simulink model "gm_inc_enc_v25"  (R2022a)
settings: Solver=FixedStepDiscrete  StartTime=0.0  StopTime=SimulationsDauer  RelTol=1e-3
undefined symbols (not defined in the file or in its folder): DiscIntNeverNeededParam, f_ISR, IncPerTurn, inital_zero_speed_timeout, n_max, OmegaPerOverSampl, Periode, Phase_Delay_A, Phase_Delay_B, PolePair, QuadratureFactor, reciprocal_iterations, T_fpga, T_mech
libraries: hdlsllib x7, hdlmdlgenlib x4, dspsrcs4 x3, dspswit3 x2, spsEdgeDetectorLib x2, simulink_extras x1
(part 2 of 2)

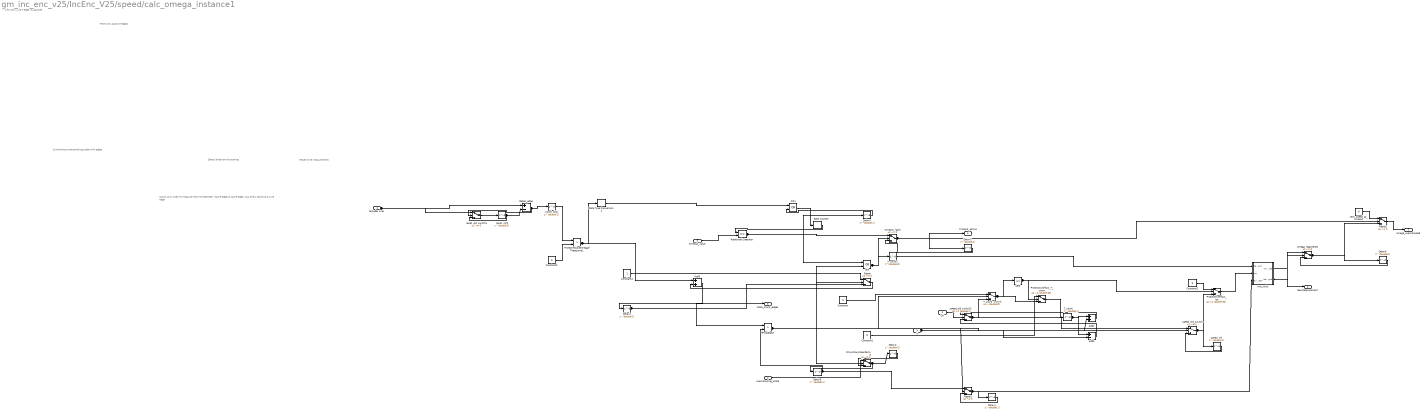
== system gm_inc_enc_v25/IncEnc_V25/speed/calc_omega_instance1 ==
  note: Count up in order to measure the time between "same edge to same edge", e.g. every positive A-Line edge
  note: Reset time measurement
  note: 1 for one cycle if edge recognized
  note: Select direction of counting
  note: Filter only positive edges
  note: Synchronize oversampling state with edges
  Encoder Line : Inport  OutDataTypeStr=boolean  PortDimensions=1  SampleTime=1e-08
  Dir : Inport  Port=2  OutDataTypeStr=fixdt(1, 4, 0)  PortDimensions=1  SampleTime=1e-08
  T : Inport  Port=3  OutDataTypeStr=fixdt(1, 38, 32)  PortDimensions=1  SampleTime=1e-08
  oversampling_state : Inport  Port=4  OutDataTypeStr=uint16  PortDimensions=1  SampleTime=1e-08
  timeout_value : Inport  Port=5  OutDataTypeStr=uint32  PortDimensions=1  SampleTime=1e-08
  32bit counter : hdlsllib/Sources/HDL Counter  CountType=Free running  CountInit=0  CountStep=1  CountMax=inital_zero_speed_timeout  CountFromType=Initial value  CountFrom=0  CountResetPort=on  CountLoadPort=off  CountEnbPort=off  CountDirPort=off  CountHitOutputPort=off  CountDataType=Unsigned  CountWordLen=32  CountFracLen=0  CountSampTime=1
  ABS : Abs  SampleTime=1e-08  OutDataTypeStr=fixdt(1, 38, 32)  SaturateOnIntegerOverflow=off
  Add1 : Sum  AccumDataTypeStr=fixdt(1, 38, 32)  OutDataTypeStr=fixdt(1, 38, 32)  SampleTime=1e-08
  Add2 : Sum  Inputs=+-  AccumDataTypeStr=fixdt(1, 38, 32)  OutDataTypeStr=fixdt(1, 38, 32)  SampleTime=1e-08
  Add3 : Sum  AccumDataTypeStr=int16  OutDataTypeStr=int16  SampleTime=1e-08
  Constant : Constant  Value=0  OutDataTypeStr=fixdt(1, 38, 32)  SampleTime=1e-08
  Constant1 : Constant  Value=0  OutDataTypeStr=fixdt(1, 38, 32)  SampleTime=1e-08
  Constant2 : Constant  Value=0  OutDataTypeStr=fixdt(1, 38, 32)  SampleTime=1e-08
  Constant3 : Constant  Value=0  OutDataTypeStr=int8  SampleTime=1e-08
  Constant4 : Constant  OutDataTypeStr=int8  SampleTime=1e-08
  Data Type Conversion1 : DataTypeConversion  OutDataTypeStr=boolean  SampleTime=1e-08  SaturateOnIntegerOverflow=off  RndMeth=Floor
  Delay{1..6,8} (7 alike) : Delay  DelayLength=double(1)  InitialCondition=0  SampleTime=1e-08
  Detec_edge : Sum  Inputs=+-  AccumDataTypeStr=int8  OutDataTypeStr=int8  SampleTime=1e-08
  IfFinalState : RelationalOperator  Operator=>  OutDataTypeStr=boolean  SampleTime=1e-08  InputSameDT=off
  OR : Logic  Operator=OR  AllPortsSameDT=off  OutDataTypeStr=boolean  SampleTime=1e-08
  OR1 : Logic  Operator=OR  AllPortsSameDT=off  OutDataTypeStr=boolean  SampleTime=1e-08
  OnlyAllowInNewPeriod : Switch  Criteria=u2 ~= 0  Threshold=double(0)  OutDataTypeStr=uint16  SampleTime=1e-08  SaturateOnIntegerOverflow=off  InputSameDT=off
  ProtectOverflow_T_count : Switch  Threshold=double(30)  OutDataTypeStr=fixdt(1, 38, 32)  SampleTime=1e-08  SaturateOnIntegerOverflow=off  InputSameDT=off
  ProtectOverflow_rps : Switch  Threshold=double(30)  OutDataTypeStr=fixdt(1, 38, 32)  SampleTime=1e-08  SaturateOnIntegerOverflow=off  InputSameDT=off
  ProtectToUseOmegaIfThetaJump1 : RelationalOperator  Operator=>  OutDataTypeStr=fixdt(1,16,0)  SampleTime=1e-08  InputSameDT=off
  Relational Operator : RelationalOperator  Operator===  OutDataTypeStr=boolean  SampleTime=1e-08  InputSameDT=off
  Reset : Switch  Criteria=u2 ~= 0  Threshold=double(0)  OutDataTypeStr=fixdt(1, 24, 11)  SampleTime=1e-08  SaturateOnIntegerOverflow=off  InputSameDT=off
  Reset1 : Switch  Criteria=u2 ~= 0  Threshold=double(0)  OutDataTypeStr=uint16  SampleTime=1e-08  SaturateOnIntegerOverflow=off  InputSameDT=off
  Reset2 : Switch  Criteria=u2 ~= 0  Threshold=double(0)  OutDataTypeStr=fixdt(1, 24, 11)  SampleTime=1e-08  SaturateOnIntegerOverflow=off  InputSameDT=off
  T_count : Delay  DelayLength=double(1)  InitialCondition=0  SampleTime=1e-08
  T_count1 : Delay  DelayLength=double(2)  InitialCondition=0  SampleTime=1e-08
  T_count_switch : Switch  Criteria=u2 > Threshold  Threshold=double(0)  OutDataTypeStr=fixdt(1, 38, 32)  SampleTime=1e-08  SaturateOnIntegerOverflow=off  InputSameDT=off
  count_old1 : Delay  DelayLength=double(1)  InitialCondition=0  SampleTime=1e-08
  invt_mult : Subsystem
  omega_registered : Switch  Criteria=u2 ~= 0  Threshold=double(0)  OutDataTypeStr=fixdt(1, 24, 11)  SampleTime=1e-08  SaturateOnIntegerOverflow=off  InputSameDT=off
  reset_old1 : Delay  DelayLength=double(1)  InitialCondition=0  SampleTime=1e-08
  reset_old_switch1 : Switch  Criteria=u2 ~= 0  Threshold=double(0)  OutDataTypeStr=boolean  SampleTime=1e-08  SaturateOnIntegerOverflow=off  InputSameDT=off
  speed_old : Delay  DelayLength=double(1)  InitialCondition=0  SampleTime=1e-08
  speed_old_switch : Switch  Criteria=u2 ~= 0  Threshold=double(0)  OutDataTypeStr=fixdt(1, 38, 32)  SampleTime=1e-08  SaturateOnIntegerOverflow=off  InputSameDT=off
  speed_old_switch2 : Switch  Threshold=double(1)  OutDataTypeStr=fixdt(1, 38, 32)  SampleTime=1e-08  SaturateOnIntegerOverflow=off  InputSameDT=off
  timeout_latch : Switch  Criteria=u2 ~= 0  Threshold=double(0)  OutDataTypeStr=boolean  SampleTime=1e-08  SaturateOnIntegerOverflow=off  InputSameDT=off
  zero_speed_at_timeout : Constant  Value=0  OutDataTypeStr=fixdt(1, 24, 11)  SampleTime=1e-08
  omega_oversampled : Outport  SampleTime=1e-08  VectorParamsAs1DForOutWhenUnconnected=off
  NewMeasurement : Outport  Port=2  SampleTime=1e-08  VectorParamsAs1DForOutWhenUnconnected=off
  state_count_edges : Outport  Port=3  SampleTime=1e-08  VectorParamsAs1DForOutWhenUnconnected=off
  timeout_active : Outport  Port=4  OutDataTypeStr=boolean  SampleTime=1e-08  VectorParamsAs1DForOutWhenUnconnected=off
  wires:
  Delay6/1 -> omega_registered/3
  Delay4/1 -> Reset1/3
  speed_old/1 -> speed_old_switch/3
  T_count_switch/1 -> ProtectOverflow_T_count/3, ABS/1
  Add1/1 -> speed_old_switch2/1
  T_count/1 -> Add2/1, Add1/1
  ProtectOverflow_T_count/1 -> T_count/1
  Add2/1 -> speed_old_switch2/3
  Delay3/1 -> timeout_latch/3
  Add3/1 -> Delay1/1
  Reset/1 -> Add3/2
  OnlyAllowInNewPeriod/1 -> Delay8/1, Delay2/1
  Delay2/1 -> OnlyAllowInNewPeriod/3
  32bit counter/1 -> Relational Operator/1
  Delay5/1 -> OR1/2
  OR1/1 -> 32bit counter/1
  reset_old1/1 -> reset_old_switch1/3, Detec_edge/2
  reset_old_switch1/1 -> reset_old1/1
  ABS/1 -> ProtectOverflow_T_count/2, ProtectOverflow_rps/2
  Constant/1 -> T_count_switch/1
  Constant1/1 -> ProtectOverflow_T_count/1
  Constant2/1 -> ProtectOverflow_rps/1
  Constant3/1 -> ProtectToUseOmegaIfThetaJump1/2
  Constant4/1 -> Reset/1
  Data Type Conversion1/1 -> OR1/1
  Delay1/1 -> Reset/3, IfFinalState/1, state_count_edges/1
  Delay8/1 -> Reset1/1, IfFinalState/2
  Detec_edge/1 -> reset_old_switch1/2, count_old1/1
  IfFinalState/1 -> Reset1/2, speed_old_switch/2, T_count_switch/2, Reset/2, OnlyAllowInNewPeriod/2, OR/2
  OR/1 -> timeout_latch/2, T_count1/1
  ProtectOverflow_rps/1 -> invt_mult/2(rps)
  ProtectToUseOmegaIfThetaJump1/1 -> Add3/1, Data Type Conversion1/1
  Relational Operator/1 -> timeout_latch/1, Delay5/1, OR/1
  Reset1/1 -> Delay4/1, invt_mult/3(Oversampling Factor)
  Reset2/1 -> omega_oversampled/1
  T_count1/1 -> invt_mult/1(New_Measurement)
  count_old1/1 -> ProtectToUseOmegaIfThetaJump1/1
  invt_mult/2(New_Measurement_delayed) -> omega_registered/2, NewMeasurement/1
  invt_mult/1(omega_oversampled) -> omega_registered/1
  omega_registered/1 -> Delay6/1, Reset2/3
  speed_old_switch/1 -> speed_old/1, ProtectOverflow_rps/3
  speed_old_switch2/1 -> speed_old_switch/1, T_count_switch/3
  timeout_latch/1 -> Delay3/1, timeout_active/1, Reset2/2
  zero_speed_at_timeout/1 -> Reset2/1
  timeout_value/1 -> Relational Operator/2
  oversampling_state/1 -> OnlyAllowInNewPeriod/1
  T/1 -> Add2/2, Add1/2
  Dir/1 -> speed_old_switch2/2
  Encoder Line/1 -> reset_old_switch1/1, Detec_edge/1

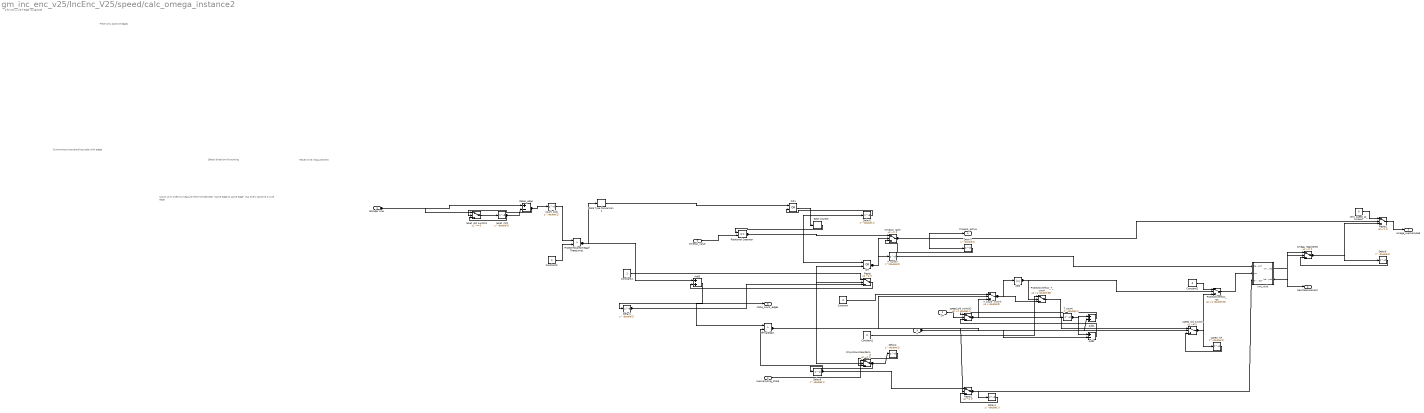
== system gm_inc_enc_v25/IncEnc_V25/speed/calc_omega_instance2 ==
  note: Count up in order to measure the time between "same edge to same edge", e.g. every positive A-Line edge
  note: Reset time measurement
  note: 1 for one cycle if edge recognized
  note: Select direction of counting
  note: Filter only positive edges
  note: Synchronize oversampling state with edges
  Encoder Line : Inport  OutDataTypeStr=boolean  PortDimensions=1  SampleTime=1e-08
  Dir : Inport  Port=2  OutDataTypeStr=fixdt(1, 4, 0)  PortDimensions=1  SampleTime=1e-08
  T : Inport  Port=3  OutDataTypeStr=fixdt(1, 38, 32)  PortDimensions=1  SampleTime=1e-08
  oversampling_state : Inport  Port=4  OutDataTypeStr=uint16  PortDimensions=1  SampleTime=1e-08
  timeout_value : Inport  Port=5  OutDataTypeStr=uint32  PortDimensions=1  SampleTime=1e-08
  32bit counter : hdlsllib/Sources/HDL Counter  CountType=Free running  CountInit=0  CountStep=1  CountMax=inital_zero_speed_timeout  CountFromType=Initial value  CountFrom=0  CountResetPort=on  CountLoadPort=off  CountEnbPort=off  CountDirPort=off  CountHitOutputPort=off  CountDataType=Unsigned  CountWordLen=32  CountFracLen=0  CountSampTime=1
  ABS : Abs  SampleTime=1e-08  OutDataTypeStr=fixdt(1, 38, 32)  SaturateOnIntegerOverflow=off
  Add1 : Sum  AccumDataTypeStr=fixdt(1, 38, 32)  OutDataTypeStr=fixdt(1, 38, 32)  SampleTime=1e-08
  Add2 : Sum  Inputs=+-  AccumDataTypeStr=fixdt(1, 38, 32)  OutDataTypeStr=fixdt(1, 38, 32)  SampleTime=1e-08
  Add3 : Sum  AccumDataTypeStr=int16  OutDataTypeStr=int16  SampleTime=1e-08
  Constant : Constant  Value=0  OutDataTypeStr=fixdt(1, 38, 32)  SampleTime=1e-08
  Constant1 : Constant  Value=0  OutDataTypeStr=fixdt(1, 38, 32)  SampleTime=1e-08
  Constant2 : Constant  Value=0  OutDataTypeStr=fixdt(1, 38, 32)  SampleTime=1e-08
  Constant3 : Constant  Value=0  OutDataTypeStr=int8  SampleTime=1e-08
  Constant4 : Constant  OutDataTypeStr=int8  SampleTime=1e-08
  Data Type Conversion1 : DataTypeConversion  OutDataTypeStr=boolean  SampleTime=1e-08  SaturateOnIntegerOverflow=off  RndMeth=Floor
  Delay{1..6,8} (7 alike) : Delay  DelayLength=double(1)  InitialCondition=0  SampleTime=1e-08
  Detec_edge : Sum  Inputs=+-  AccumDataTypeStr=int8  OutDataTypeStr=int8  SampleTime=1e-08
  IfFinalState : RelationalOperator  Operator=>  OutDataTypeStr=boolean  SampleTime=1e-08  InputSameDT=off
  OR : Logic  Operator=OR  AllPortsSameDT=off  OutDataTypeStr=boolean  SampleTime=1e-08
  OR1 : Logic  Operator=OR  AllPortsSameDT=off  OutDataTypeStr=boolean  SampleTime=1e-08
  OnlyAllowInNewPeriod : Switch  Criteria=u2 ~= 0  Threshold=double(0)  OutDataTypeStr=uint16  SampleTime=1e-08  SaturateOnIntegerOverflow=off  InputSameDT=off
  ProtectOverflow_T_count : Switch  Threshold=double(30)  OutDataTypeStr=fixdt(1, 38, 32)  SampleTime=1e-08  SaturateOnIntegerOverflow=off  InputSameDT=off
  ProtectOverflow_rps : Switch  Threshold=double(30)  OutDataTypeStr=fixdt(1, 38, 32)  SampleTime=1e-08  SaturateOnIntegerOverflow=off  InputSameDT=off
  ProtectToUseOmegaIfThetaJump1 : RelationalOperator  Operator=>  OutDataTypeStr=fixdt(1,16,0)  SampleTime=1e-08  InputSameDT=off
  Relational Operator : RelationalOperator  Operator===  OutDataTypeStr=boolean  SampleTime=1e-08  InputSameDT=off
  Reset : Switch  Criteria=u2 ~= 0  Threshold=double(0)  OutDataTypeStr=fixdt(1, 24, 11)  SampleTime=1e-08  SaturateOnIntegerOverflow=off  InputSameDT=off
  Reset1 : Switch  Criteria=u2 ~= 0  Threshold=double(0)  OutDataTypeStr=uint16  SampleTime=1e-08  SaturateOnIntegerOverflow=off  InputSameDT=off
  Reset2 : Switch  Criteria=u2 ~= 0  Threshold=double(0)  OutDataTypeStr=fixdt(1, 24, 11)  SampleTime=1e-08  SaturateOnIntegerOverflow=off  InputSameDT=off
  T_count : Delay  DelayLength=double(1)  InitialCondition=0  SampleTime=1e-08
  T_count1 : Delay  DelayLength=double(2)  InitialCondition=0  SampleTime=1e-08
  T_count_switch : Switch  Criteria=u2 > Threshold  Threshold=double(0)  OutDataTypeStr=fixdt(1, 38, 32)  SampleTime=1e-08  SaturateOnIntegerOverflow=off  InputSameDT=off
  count_old1 : Delay  DelayLength=double(1)  InitialCondition=0  SampleTime=1e-08
  invt_mult : Subsystem
  omega_registered : Switch  Criteria=u2 ~= 0  Threshold=double(0)  OutDataTypeStr=fixdt(1, 24, 11)  SampleTime=1e-08  SaturateOnIntegerOverflow=off  InputSameDT=off
  reset_old1 : Delay  DelayLength=double(1)  InitialCondition=0  SampleTime=1e-08
  reset_old_switch1 : Switch  Criteria=u2 ~= 0  Threshold=double(0)  OutDataTypeStr=boolean  SampleTime=1e-08  SaturateOnIntegerOverflow=off  InputSameDT=off
  speed_old : Delay  DelayLength=double(1)  InitialCondition=0  SampleTime=1e-08
  speed_old_switch : Switch  Criteria=u2 ~= 0  Threshold=double(0)  OutDataTypeStr=fixdt(1, 38, 32)  SampleTime=1e-08  SaturateOnIntegerOverflow=off  InputSameDT=off
  speed_old_switch2 : Switch  Threshold=double(1)  OutDataTypeStr=fixdt(1, 38, 32)  SampleTime=1e-08  SaturateOnIntegerOverflow=off  InputSameDT=off
  timeout_latch : Switch  Criteria=u2 ~= 0  Threshold=double(0)  OutDataTypeStr=boolean  SampleTime=1e-08  SaturateOnIntegerOverflow=off  InputSameDT=off
  zero_speed_at_timeout : Constant  Value=0  OutDataTypeStr=fixdt(1, 24, 11)  SampleTime=1e-08
  omega_oversampled : Outport  SampleTime=1e-08  VectorParamsAs1DForOutWhenUnconnected=off
  NewMeasurement : Outport  Port=2  SampleTime=1e-08  VectorParamsAs1DForOutWhenUnconnected=off
  state_count_edges : Outport  Port=3  SampleTime=1e-08  VectorParamsAs1DForOutWhenUnconnected=off
  timeout_active : Outport  Port=4  OutDataTypeStr=boolean  SampleTime=1e-08  VectorParamsAs1DForOutWhenUnconnected=off
  wires:
  Delay6/1 -> omega_registered/3
  Delay4/1 -> Reset1/3
  speed_old/1 -> speed_old_switch/3
  T_count_switch/1 -> ProtectOverflow_T_count/3, ABS/1
  Add1/1 -> speed_old_switch2/1
  T_count/1 -> Add2/1, Add1/1
  ProtectOverflow_T_count/1 -> T_count/1
  Add2/1 -> speed_old_switch2/3
  Delay3/1 -> timeout_latch/3
  Add3/1 -> Delay1/1
  Reset/1 -> Add3/2
  OnlyAllowInNewPeriod/1 -> Delay8/1, Delay2/1
  Delay2/1 -> OnlyAllowInNewPeriod/3
  32bit counter/1 -> Relational Operator/1
  Delay5/1 -> OR1/2
  OR1/1 -> 32bit counter/1
  reset_old1/1 -> reset_old_switch1/3, Detec_edge/2
  reset_old_switch1/1 -> reset_old1/1
  ABS/1 -> ProtectOverflow_T_count/2, ProtectOverflow_rps/2
  Constant/1 -> T_count_switch/1
  Constant1/1 -> ProtectOverflow_T_count/1
  Constant2/1 -> ProtectOverflow_rps/1
  Constant3/1 -> ProtectToUseOmegaIfThetaJump1/2
  Constant4/1 -> Reset/1
  Data Type Conversion1/1 -> OR1/1
  Delay1/1 -> Reset/3, IfFinalState/1, state_count_edges/1
  Delay8/1 -> Reset1/1, IfFinalState/2
  Detec_edge/1 -> reset_old_switch1/2, count_old1/1
  IfFinalState/1 -> Reset1/2, speed_old_switch/2, T_count_switch/2, Reset/2, OnlyAllowInNewPeriod/2, OR/2
  OR/1 -> timeout_latch/2, T_count1/1
  ProtectOverflow_rps/1 -> invt_mult/2(rps)
  ProtectToUseOmegaIfThetaJump1/1 -> Add3/1, Data Type Conversion1/1
  Relational Operator/1 -> timeout_latch/1, Delay5/1, OR/1
  Reset1/1 -> Delay4/1, invt_mult/3(Oversampling Factor)
  Reset2/1 -> omega_oversampled/1
  T_count1/1 -> invt_mult/1(New_Measurement)
  count_old1/1 -> ProtectToUseOmegaIfThetaJump1/1
  invt_mult/2(New_Measurement_delayed) -> omega_registered/2, NewMeasurement/1
  invt_mult/1(omega_oversampled) -> omega_registered/1
  omega_registered/1 -> Delay6/1, Reset2/3
  speed_old_switch/1 -> speed_old/1, ProtectOverflow_rps/3
  speed_old_switch2/1 -> speed_old_switch/1, T_count_switch/3
  timeout_latch/1 -> Delay3/1, timeout_active/1, Reset2/2
  zero_speed_at_timeout/1 -> Reset2/1
  timeout_value/1 -> Relational Operator/2
  oversampling_state/1 -> OnlyAllowInNewPeriod/1
  T/1 -> Add2/2, Add1/2
  Dir/1 -> speed_old_switch2/2
  Encoder Line/1 -> reset_old_switch1/1, Detec_edge/1

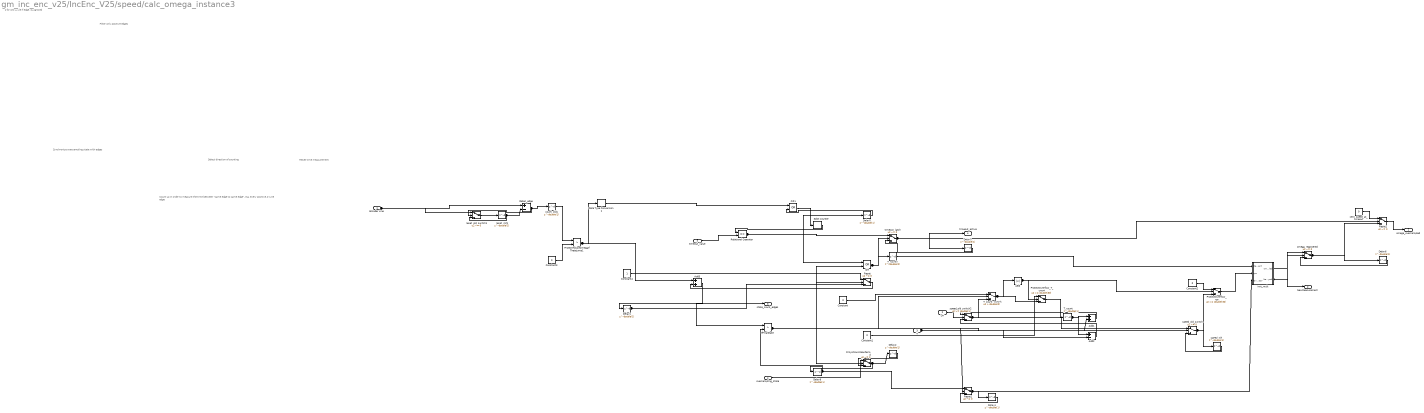
== system gm_inc_enc_v25/IncEnc_V25/speed/calc_omega_instance3 ==
  note: Count up in order to measure the time between "same edge to same edge", e.g. every positive A-Line edge
  note: Reset time measurement
  note: 1 for one cycle if edge recognized
  note: Select direction of counting
  note: Filter only positive edges
  note: Synchronize oversampling state with edges
  Encoder Line : Inport  OutDataTypeStr=boolean  PortDimensions=1  SampleTime=1e-08
  Dir : Inport  Port=2  OutDataTypeStr=fixdt(1, 4, 0)  PortDimensions=1  SampleTime=1e-08
  T : Inport  Port=3  OutDataTypeStr=fixdt(1, 38, 32)  PortDimensions=1  SampleTime=1e-08
  oversampling_state : Inport  Port=4  OutDataTypeStr=uint16  PortDimensions=1  SampleTime=1e-08
  timeout_value : Inport  Port=5  OutDataTypeStr=uint32  PortDimensions=1  SampleTime=1e-08
  32bit counter : hdlsllib/Sources/HDL Counter  CountType=Free running  CountInit=0  CountStep=1  CountMax=inital_zero_speed_timeout  CountFromType=Initial value  CountFrom=0  CountResetPort=on  CountLoadPort=off  CountEnbPort=off  CountDirPort=off  CountHitOutputPort=off  CountDataType=Unsigned  CountWordLen=32  CountFracLen=0  CountSampTime=1
  ABS : Abs  SampleTime=1e-08  OutDataTypeStr=fixdt(1, 38, 32)  SaturateOnIntegerOverflow=off
  Add1 : Sum  AccumDataTypeStr=fixdt(1, 38, 32)  OutDataTypeStr=fixdt(1, 38, 32)  SampleTime=1e-08
  Add2 : Sum  Inputs=+-  AccumDataTypeStr=fixdt(1, 38, 32)  OutDataTypeStr=fixdt(1, 38, 32)  SampleTime=1e-08
  Add3 : Sum  AccumDataTypeStr=int16  OutDataTypeStr=int16  SampleTime=1e-08
  Constant : Constant  Value=0  OutDataTypeStr=fixdt(1, 38, 32)  SampleTime=1e-08
  Constant1 : Constant  Value=0  OutDataTypeStr=fixdt(1, 38, 32)  SampleTime=1e-08
  Constant2 : Constant  Value=0  OutDataTypeStr=fixdt(1, 38, 32)  SampleTime=1e-08
  Constant3 : Constant  Value=0  OutDataTypeStr=int8  SampleTime=1e-08
  Constant4 : Constant  OutDataTypeStr=int8  SampleTime=1e-08
  Data Type Conversion1 : DataTypeConversion  OutDataTypeStr=boolean  SampleTime=1e-08  SaturateOnIntegerOverflow=off  RndMeth=Floor
  Delay{1..6,8} (7 alike) : Delay  DelayLength=double(1)  InitialCondition=0  SampleTime=1e-08
  Detec_edge : Sum  Inputs=+-  AccumDataTypeStr=int8  OutDataTypeStr=int8  SampleTime=1e-08
  IfFinalState : RelationalOperator  Operator=>  OutDataTypeStr=boolean  SampleTime=1e-08  InputSameDT=off
  OR : Logic  Operator=OR  AllPortsSameDT=off  OutDataTypeStr=boolean  SampleTime=1e-08
  OR1 : Logic  Operator=OR  AllPortsSameDT=off  OutDataTypeStr=boolean  SampleTime=1e-08
  OnlyAllowInNewPeriod : Switch  Criteria=u2 ~= 0  Threshold=double(0)  OutDataTypeStr=uint16  SampleTime=1e-08  SaturateOnIntegerOverflow=off  InputSameDT=off
  ProtectOverflow_T_count : Switch  Threshold=double(30)  OutDataTypeStr=fixdt(1, 38, 32)  SampleTime=1e-08  SaturateOnIntegerOverflow=off  InputSameDT=off
  ProtectOverflow_rps : Switch  Threshold=double(30)  OutDataTypeStr=fixdt(1, 38, 32)  SampleTime=1e-08  SaturateOnIntegerOverflow=off  InputSameDT=off
  ProtectToUseOmegaIfThetaJump1 : RelationalOperator  Operator=>  OutDataTypeStr=fixdt(1,16,0)  SampleTime=1e-08  InputSameDT=off
  Relational Operator : RelationalOperator  Operator===  OutDataTypeStr=boolean  SampleTime=1e-08  InputSameDT=off
  Reset : Switch  Criteria=u2 ~= 0  Threshold=double(0)  OutDataTypeStr=fixdt(1, 24, 11)  SampleTime=1e-08  SaturateOnIntegerOverflow=off  InputSameDT=off
  Reset1 : Switch  Criteria=u2 ~= 0  Threshold=double(0)  OutDataTypeStr=uint16  SampleTime=1e-08  SaturateOnIntegerOverflow=off  InputSameDT=off
  Reset2 : Switch  Criteria=u2 ~= 0  Threshold=double(0)  OutDataTypeStr=fixdt(1, 24, 11)  SampleTime=1e-08  SaturateOnIntegerOverflow=off  InputSameDT=off
  T_count : Delay  DelayLength=double(1)  InitialCondition=0  SampleTime=1e-08
  T_count1 : Delay  DelayLength=double(2)  InitialCondition=0  SampleTime=1e-08
  T_count_switch : Switch  Criteria=u2 > Threshold  Threshold=double(0)  OutDataTypeStr=fixdt(1, 38, 32)  SampleTime=1e-08  SaturateOnIntegerOverflow=off  InputSameDT=off
  count_old1 : Delay  DelayLength=double(1)  InitialCondition=0  SampleTime=1e-08
  invt_mult : Subsystem
  omega_registered : Switch  Criteria=u2 ~= 0  Threshold=double(0)  OutDataTypeStr=fixdt(1, 24, 11)  SampleTime=1e-08  SaturateOnIntegerOverflow=off  InputSameDT=off
  reset_old1 : Delay  DelayLength=double(1)  InitialCondition=0  SampleTime=1e-08
  reset_old_switch1 : Switch  Criteria=u2 ~= 0  Threshold=double(0)  OutDataTypeStr=boolean  SampleTime=1e-08  SaturateOnIntegerOverflow=off  InputSameDT=off
  speed_old : Delay  DelayLength=double(1)  InitialCondition=0  SampleTime=1e-08
  speed_old_switch : Switch  Criteria=u2 ~= 0  Threshold=double(0)  OutDataTypeStr=fixdt(1, 38, 32)  SampleTime=1e-08  SaturateOnIntegerOverflow=off  InputSameDT=off
  speed_old_switch2 : Switch  Threshold=double(1)  OutDataTypeStr=fixdt(1, 38, 32)  SampleTime=1e-08  SaturateOnIntegerOverflow=off  InputSameDT=off
  timeout_latch : Switch  Criteria=u2 ~= 0  Threshold=double(0)  OutDataTypeStr=boolean  SampleTime=1e-08  SaturateOnIntegerOverflow=off  InputSameDT=off
  zero_speed_at_timeout : Constant  Value=0  OutDataTypeStr=fixdt(1, 24, 11)  SampleTime=1e-08
  omega_oversampled : Outport  SampleTime=1e-08  VectorParamsAs1DForOutWhenUnconnected=off
  NewMeasurement : Outport  Port=2  SampleTime=1e-08  VectorParamsAs1DForOutWhenUnconnected=off
  state_count_edges : Outport  Port=3  SampleTime=1e-08  VectorParamsAs1DForOutWhenUnconnected=off
  timeout_active : Outport  Port=4  OutDataTypeStr=boolean  SampleTime=1e-08  VectorParamsAs1DForOutWhenUnconnected=off
  wires:
  Delay6/1 -> omega_registered/3
  Delay4/1 -> Reset1/3
  speed_old/1 -> speed_old_switch/3
  T_count_switch/1 -> ProtectOverflow_T_count/3, ABS/1
  Add1/1 -> speed_old_switch2/1
  T_count/1 -> Add2/1, Add1/1
  ProtectOverflow_T_count/1 -> T_count/1
  Add2/1 -> speed_old_switch2/3
  Delay3/1 -> timeout_latch/3
  Add3/1 -> Delay1/1
  Reset/1 -> Add3/2
  OnlyAllowInNewPeriod/1 -> Delay8/1, Delay2/1
  Delay2/1 -> OnlyAllowInNewPeriod/3
  32bit counter/1 -> Relational Operator/1
  Delay5/1 -> OR1/2
  OR1/1 -> 32bit counter/1
  reset_old1/1 -> reset_old_switch1/3, Detec_edge/2
  reset_old_switch1/1 -> reset_old1/1
  ABS/1 -> ProtectOverflow_T_count/2, ProtectOverflow_rps/2
  Constant/1 -> T_count_switch/1
  Constant1/1 -> ProtectOverflow_T_count/1
  Constant2/1 -> ProtectOverflow_rps/1
  Constant3/1 -> ProtectToUseOmegaIfThetaJump1/2
  Constant4/1 -> Reset/1
  Data Type Conversion1/1 -> OR1/1
  Delay1/1 -> Reset/3, IfFinalState/1, state_count_edges/1
  Delay8/1 -> Reset1/1, IfFinalState/2
  Detec_edge/1 -> reset_old_switch1/2, count_old1/1
  IfFinalState/1 -> Reset1/2, speed_old_switch/2, T_count_switch/2, Reset/2, OnlyAllowInNewPeriod/2, OR/2
  OR/1 -> timeout_latch/2, T_count1/1
  ProtectOverflow_rps/1 -> invt_mult/2(rps)
  ProtectToUseOmegaIfThetaJump1/1 -> Add3/1, Data Type Conversion1/1
  Relational Operator/1 -> timeout_latch/1, Delay5/1, OR/1
  Reset1/1 -> Delay4/1, invt_mult/3(Oversampling Factor)
  Reset2/1 -> omega_oversampled/1
  T_count1/1 -> invt_mult/1(New_Measurement)
  count_old1/1 -> ProtectToUseOmegaIfThetaJump1/1
  invt_mult/2(New_Measurement_delayed) -> omega_registered/2, NewMeasurement/1
  invt_mult/1(omega_oversampled) -> omega_registered/1
  omega_registered/1 -> Delay6/1, Reset2/3
  speed_old_switch/1 -> speed_old/1, ProtectOverflow_rps/3
  speed_old_switch2/1 -> speed_old_switch/1, T_count_switch/3
  timeout_latch/1 -> Delay3/1, timeout_active/1, Reset2/2
  zero_speed_at_timeout/1 -> Reset2/1
  timeout_value/1 -> Relational Operator/2
  oversampling_state/1 -> OnlyAllowInNewPeriod/1
  T/1 -> Add2/2, Add1/2
  Dir/1 -> speed_old_switch2/2
  Encoder Line/1 -> reset_old_switch1/1, Detec_edge/1

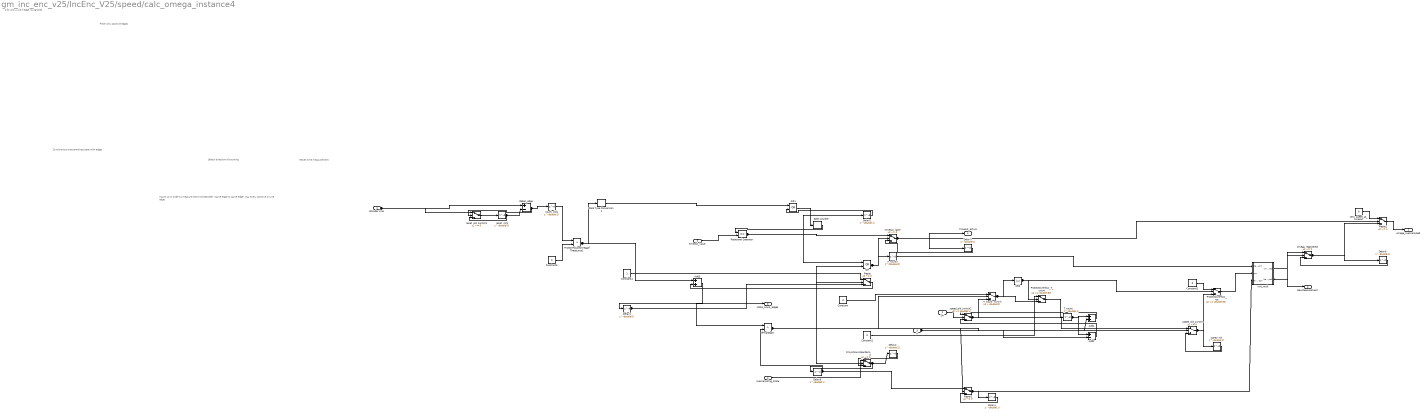
== system gm_inc_enc_v25/IncEnc_V25/speed/calc_omega_instance4 ==
  note: Synchronize oversampling state with edges
  note: Filter only positive edges
  note: Select direction of counting
  note: 1 for one cycle if edge recognized
  note: Reset time measurement
  note: Count up in order to measure the time between "same edge to same edge", e.g. every positive A-Line edge
  Encoder Line : Inport  OutDataTypeStr=boolean  PortDimensions=1  SampleTime=1e-08
  Dir : Inport  Port=2  OutDataTypeStr=fixdt(1, 4, 0)  PortDimensions=1  SampleTime=1e-08
  T : Inport  Port=3  OutDataTypeStr=fixdt(1, 38, 32)  PortDimensions=1  SampleTime=1e-08
  oversampling_state : Inport  Port=4  OutDataTypeStr=uint16  PortDimensions=1  SampleTime=1e-08
  timeout_value : Inport  Port=5  OutDataTypeStr=uint32  PortDimensions=1  SampleTime=1e-08
  32bit counter : hdlsllib/Sources/HDL Counter  CountType=Free running  CountInit=0  CountStep=1  CountMax=inital_zero_speed_timeout  CountFromType=Initial value  CountFrom=0  CountResetPort=on  CountLoadPort=off  CountEnbPort=off  CountDirPort=off  CountHitOutputPort=off  CountDataType=Unsigned  CountWordLen=32  CountFracLen=0  CountSampTime=1
  ABS : Abs  SampleTime=1e-08  OutDataTypeStr=fixdt(1, 38, 32)  SaturateOnIntegerOverflow=off
  Add1 : Sum  AccumDataTypeStr=fixdt(1, 38, 32)  OutDataTypeStr=fixdt(1, 38, 32)  SampleTime=1e-08
  Add2 : Sum  Inputs=+-  AccumDataTypeStr=fixdt(1, 38, 32)  OutDataTypeStr=fixdt(1, 38, 32)  SampleTime=1e-08
  Add3 : Sum  AccumDataTypeStr=int16  OutDataTypeStr=int16  SampleTime=1e-08
  Constant : Constant  Value=0  OutDataTypeStr=fixdt(1, 38, 32)  SampleTime=1e-08
  Constant1 : Constant  Value=0  OutDataTypeStr=fixdt(1, 38, 32)  SampleTime=1e-08
  Constant2 : Constant  Value=0  OutDataTypeStr=fixdt(1, 38, 32)  SampleTime=1e-08
  Constant3 : Constant  Value=0  OutDataTypeStr=int8  SampleTime=1e-08
  Constant4 : Constant  OutDataTypeStr=int8  SampleTime=1e-08
  Data Type Conversion1 : DataTypeConversion  OutDataTypeStr=boolean  SampleTime=1e-08  SaturateOnIntegerOverflow=off  RndMeth=Floor
  Delay{1..6,8} (7 alike) : Delay  DelayLength=double(1)  InitialCondition=0  SampleTime=1e-08
  Detec_edge : Sum  Inputs=+-  AccumDataTypeStr=int8  OutDataTypeStr=int8  SampleTime=1e-08
  IfFinalState : RelationalOperator  Operator=>  OutDataTypeStr=boolean  SampleTime=1e-08  InputSameDT=off
  OR : Logic  Operator=OR  AllPortsSameDT=off  OutDataTypeStr=boolean  SampleTime=1e-08
  OR1 : Logic  Operator=OR  AllPortsSameDT=off  OutDataTypeStr=boolean  SampleTime=1e-08
  OnlyAllowInNewPeriod : Switch  Criteria=u2 ~= 0  Threshold=double(0)  OutDataTypeStr=uint16  SampleTime=1e-08  SaturateOnIntegerOverflow=off  InputSameDT=off
  ProtectOverflow_T_count : Switch  Threshold=double(30)  OutDataTypeStr=fixdt(1, 38, 32)  SampleTime=1e-08  SaturateOnIntegerOverflow=off  InputSameDT=off
  ProtectOverflow_rps : Switch  Threshold=double(30)  OutDataTypeStr=fixdt(1, 38, 32)  SampleTime=1e-08  SaturateOnIntegerOverflow=off  InputSameDT=off
  ProtectToUseOmegaIfThetaJump1 : RelationalOperator  Operator=>  OutDataTypeStr=fixdt(1,16,0)  SampleTime=1e-08  InputSameDT=off
  Relational Operator : RelationalOperator  Operator===  OutDataTypeStr=boolean  SampleTime=1e-08  InputSameDT=off
  Reset : Switch  Criteria=u2 ~= 0  Threshold=double(0)  OutDataTypeStr=fixdt(1, 24, 11)  SampleTime=1e-08  SaturateOnIntegerOverflow=off  InputSameDT=off
  Reset1 : Switch  Criteria=u2 ~= 0  Threshold=double(0)  OutDataTypeStr=uint16  SampleTime=1e-08  SaturateOnIntegerOverflow=off  InputSameDT=off
  Reset2 : Switch  Criteria=u2 ~= 0  Threshold=double(0)  OutDataTypeStr=fixdt(1, 24, 11)  SampleTime=1e-08  SaturateOnIntegerOverflow=off  InputSameDT=off
  T_count : Delay  DelayLength=double(1)  InitialCondition=0  SampleTime=1e-08
  T_count1 : Delay  DelayLength=double(2)  InitialCondition=0  SampleTime=1e-08
  T_count_switch : Switch  Criteria=u2 > Threshold  Threshold=double(0)  OutDataTypeStr=fixdt(1, 38, 32)  SampleTime=1e-08  SaturateOnIntegerOverflow=off  InputSameDT=off
  count_old1 : Delay  DelayLength=double(1)  InitialCondition=0  SampleTime=1e-08
  invt_mult : Subsystem
  omega_registered : Switch  Criteria=u2 ~= 0  Threshold=double(0)  OutDataTypeStr=fixdt(1, 24, 11)  SampleTime=1e-08  SaturateOnIntegerOverflow=off  InputSameDT=off
  reset_old1 : Delay  DelayLength=double(1)  InitialCondition=0  SampleTime=1e-08
  reset_old_switch1 : Switch  Criteria=u2 ~= 0  Threshold=double(0)  OutDataTypeStr=boolean  SampleTime=1e-08  SaturateOnIntegerOverflow=off  InputSameDT=off
  speed_old : Delay  DelayLength=double(1)  InitialCondition=0  SampleTime=1e-08
  speed_old_switch : Switch  Criteria=u2 ~= 0  Threshold=double(0)  OutDataTypeStr=fixdt(1, 38, 32)  SampleTime=1e-08  SaturateOnIntegerOverflow=off  InputSameDT=off
  speed_old_switch2 : Switch  Threshold=double(1)  OutDataTypeStr=fixdt(1, 38, 32)  SampleTime=1e-08  SaturateOnIntegerOverflow=off  InputSameDT=off
  timeout_latch : Switch  Criteria=u2 ~= 0  Threshold=double(0)  OutDataTypeStr=boolean  SampleTime=1e-08  SaturateOnIntegerOverflow=off  InputSameDT=off
  zero_speed_at_timeout : Constant  Value=0  OutDataTypeStr=fixdt(1, 24, 11)  SampleTime=1e-08
  omega_oversampled : Outport  SampleTime=1e-08  VectorParamsAs1DForOutWhenUnconnected=off
  NewMeasurement : Outport  Port=2  SampleTime=1e-08  VectorParamsAs1DForOutWhenUnconnected=off
  state_count_edges : Outport  Port=3  SampleTime=1e-08  VectorParamsAs1DForOutWhenUnconnected=off
  timeout_active : Outport  Port=4  OutDataTypeStr=boolean  SampleTime=1e-08  VectorParamsAs1DForOutWhenUnconnected=off
  wires:
  Encoder Line/1 -> Detec_edge/1, reset_old_switch1/1
  Dir/1 -> speed_old_switch2/2
  T/1 -> Add1/2, Add2/2
  oversampling_state/1 -> OnlyAllowInNewPeriod/1
  timeout_value/1 -> Relational Operator/2
  zero_speed_at_timeout/1 -> Reset2/1
  timeout_latch/1 -> Reset2/2, timeout_active/1, Delay3/1
  speed_old_switch2/1 -> T_count_switch/3, speed_old_switch/1
  speed_old_switch/1 -> ProtectOverflow_rps/3, speed_old/1
  omega_registered/1 -> Reset2/3, Delay6/1
  invt_mult/1(omega_oversampled) -> omega_registered/1
  invt_mult/2(New_Measurement_delayed) -> NewMeasurement/1, omega_registered/2
  count_old1/1 -> ProtectToUseOmegaIfThetaJump1/1
  T_count1/1 -> invt_mult/1(New_Measurement)
  Reset2/1 -> omega_oversampled/1
  Reset1/1 -> invt_mult/3(Oversampling Factor), Delay4/1
  Relational Operator/1 -> OR/1, Delay5/1, timeout_latch/1
  ProtectToUseOmegaIfThetaJump1/1 -> Data Type Conversion1/1, Add3/1
  ProtectOverflow_rps/1 -> invt_mult/2(rps)
  OR/1 -> T_count1/1, timeout_latch/2
  IfFinalState/1 -> OR/2, OnlyAllowInNewPeriod/2, Reset/2, T_count_switch/2, speed_old_switch/2, Reset1/2
  Detec_edge/1 -> count_old1/1, reset_old_switch1/2
  Delay8/1 -> IfFinalState/2, Reset1/1
  Delay1/1 -> state_count_edges/1, IfFinalState/1, Reset/3
  Data Type Conversion1/1 -> OR1/1
  Constant4/1 -> Reset/1
  Constant3/1 -> ProtectToUseOmegaIfThetaJump1/2
  Constant2/1 -> ProtectOverflow_rps/1
  Constant1/1 -> ProtectOverflow_T_count/1
  Constant/1 -> T_count_switch/1
  ABS/1 -> ProtectOverflow_rps/2, ProtectOverflow_T_count/2
  reset_old_switch1/1 -> reset_old1/1
  reset_old1/1 -> Detec_edge/2, reset_old_switch1/3
  OR1/1 -> 32bit counter/1
  Delay5/1 -> OR1/2
  32bit counter/1 -> Relational Operator/1
  Delay2/1 -> OnlyAllowInNewPeriod/3
  OnlyAllowInNewPeriod/1 -> Delay2/1, Delay8/1
  Reset/1 -> Add3/2
  Add3/1 -> Delay1/1
  Delay3/1 -> timeout_latch/3
  Add2/1 -> speed_old_switch2/3
  ProtectOverflow_T_count/1 -> T_count/1
  T_count/1 -> Add1/1, Add2/1
  Add1/1 -> speed_old_switch2/1
  T_count_switch/1 -> ABS/1, ProtectOverflow_T_count/3
  speed_old/1 -> speed_old_switch/3
  Delay4/1 -> Reset1/3
  Delay6/1 -> omega_registered/3

== system gm_inc_enc_v25/IncrementalEncoder_Floating/n_aus_theta_v4/Geschwindigkeitsfilter1 ==
  In1 : Inport
  Add1 : Sum  Inputs=+-
  Discrete-Time Integrator2 : DiscreteIntegrator  SampleTime=-1  ICPrevOutput=DiscIntNeverNeededParam  ICPrevScaledInput=DiscIntNeverNeededParam
  Gain2 2500 10000 : Gain  Gain=10000
  Scope1 : Scope  NumInputPorts=5
  Out1 : Outport  InitialOutput=[0]  VectorParamsAs1DForOutWhenUnconnected=off
  wires:
  In1/1 -> Add1/1, Scope1/5
  Discrete-Time Integrator2/1 -> Add1/2, Out1/1, Scope1/2
  Gain2 2500 10000/1 -> Discrete-Time Integrator2/1, Scope1/3
  Add1/1 -> Gain2 2500 10000/1, Scope1/4

== system gm_inc_enc_v25/IncEnc_V25/speed/OS_factor_logic/align_oversamples ==
  oversampling_factor : Inport  OutDataTypeStr=uint16  PortDimensions=1  SampleTime=1e-08
  new_transition : Inport  Port=2  OutDataTypeStr=boolean  PortDimensions=[4]  SampleTime=1e-08
  states : Inport  Port=3  OutDataTypeStr=int16  PortDimensions=[4]  SampleTime=1e-08
  align_oversamples : MATLAB Function  TreatAsAtomicUnit=on
  delay_output : Outport  SampleTime=1e-08  VectorParamsAs1DForOutWhenUnconnected=off
  wires:
  oversampling_factor/1 -> align_oversamples/1(oversampling_factor)
  new_transition/1 -> align_oversamples/2(new_transition)
  states/1 -> align_oversamples/3(states)
  align_oversamples/1(delay_output) -> delay_output/1

== system gm_inc_enc_v25/IncEnc_V25/speed/OS_factor_logic/oversample_factor ==
  AllowCheckOverSampl : Inport  OutDataTypeStr=boolean  PortDimensions=1  SampleTime=1e-08
  ReadBack_Omega : Inport  Port=2  OutDataTypeStr=fixdt(1, 24, 11)  PortDimensions=1  SampleTime=1e-08
  OverSamplOmega : Inport  Port=3  OutDataTypeStr=fixdt(1, 24, 11)  PortDimensions=1  SampleTime=1e-08
  state : Inport  Port=4  OutDataTypeStr=uint16  PortDimensions=1  SampleTime=1e-08
  InternalOmega : Inport  Port=5  OutDataTypeStr=fixdt(1, 24, 11)  PortDimensions=1  SampleTime=1e-08
  oversample_factor : MATLAB Function  TreatAsAtomicUnit=on
  state_Out : Outport  SampleTime=1e-08  VectorParamsAs1DForOutWhenUnconnected=off
  InternalOmega_Out : Outport  Port=2  SampleTime=1e-08  VectorParamsAs1DForOutWhenUnconnected=off
  wires:
  AllowCheckOverSampl/1 -> oversample_factor/1(AllowCheckOverSampl)
  ReadBack_Omega/1 -> oversample_factor/2(ReadBack_Omega)
  OverSamplOmega/1 -> oversample_factor/3(OverSamplOmega)
  state/1 -> oversample_factor/4(state)
  InternalOmega/1 -> oversample_factor/5(InternalOmega)
  oversample_factor/1(state_Out) -> state_Out/1
  oversample_factor/2(InternalOmega_Out) -> InternalOmega_Out/1

== system gm_inc_enc_v25/IncEnc_V25/speed/calc_omega_instance1/invt_mult ==
  note: Invert 1/omega and muliply with synchronized oversampling factor
  New_Measurement : Inport  OutDataTypeStr=boolean  PortDimensions=1  SampleTime=1e-08
  rps : Inport  Port=2  OutDataTypeStr=fixdt(1, 38, 32)  PortDimensions=1  SampleTime=1e-08
  Oversampling Factor : Inport  Port=3  OutDataTypeStr=uint16  PortDimensions=1  SampleTime=1e-08
  Data Type Conversion2 : DataTypeConversion  OutDataTypeStr=fixdt(1, 24, 12)  SampleTime=1e-08  SaturateOnIntegerOverflow=off  RndMeth=Floor
  Data Type Conversion3 : DataTypeConversion  OutDataTypeStr=fixdt(0, 6, 0)  SampleTime=1e-08  SaturateOnIntegerOverflow=off  RndMeth=Floor
  Data Type Conversion4 : DataTypeConversion  OutDataTypeStr=fixdt(1, 32, 18)  SampleTime=1e-08  SaturateOnIntegerOverflow=off  RndMeth=Floor
  Div_i1 : Product  Inputs=**  OutDataTypeStr=fixdt(1, 30, 12)  SampleTime=1e-08
  Div_i1_out_dtc : DataTypeConversion  OutDataTypeStr=fixdt(1, 24, 11)  RndMeth=Simplest  SampleTime=1e-08
  HDL Reciprocal : Subsystem
  delayMatch : Delay  DelayLength=double(9)  InitialCondition=0  SampleTime=1e-08
  in_0_pipe : Delay  DelayLength=double(1)  InitialCondition=0  SampleTime=1e-08
  in_1_pipe : Delay  DelayLength=double(1)  InitialCondition=0  SampleTime=1e-08
  out_1_pipe : Delay  DelayLength=double(1)  InitialCondition=0  SampleTime=1e-08
  rd_{0..1,3..4} (4 alike) : Delay  DelayLength=double(1)  InitialCondition=0  SampleTime=1e-08
  rd_2 : Delay  DelayLength=double(8)  InitialCondition=0  SampleTime=1e-08
  omega_oversampled : Outport  SampleTime=1e-08
  New_Measurement_delayed : Outport  Port=2  SampleTime=1e-08
  wires:
  in_1_pipe/1 -> Data Type Conversion4/1
  out_1_pipe/1 -> delayMatch/1
  in_0_pipe/1 -> out_1_pipe/1
  Div_i1_out_dtc/1 -> rd_4/1
  rd_3/1 -> Div_i1_out_dtc/1
  Div_i1/1 -> rd_3/1
  rd_2/1 -> Div_i1/2
  Data Type Conversion3/1 -> rd_2/1
  Data Type Conversion2/1 -> Div_i1/1
  rd_1/1 -> Data Type Conversion3/1
  rd_0/1 -> Data Type Conversion2/1
  Oversampling Factor/1 -> rd_1/1
  rps/1 -> in_1_pipe/1
  New_Measurement/1 -> in_0_pipe/1
  HDL Reciprocal/1(Out1) -> rd_0/1
  delayMatch/1 -> New_Measurement_delayed/1
  rd_4/1 -> omega_oversampled/1
  Data Type Conversion4/1 -> HDL Reciprocal/1(In1)

== system gm_inc_enc_v25/IncEnc_V25/speed/calc_omega_instance2/invt_mult ==
  note: Invert 1/omega and muliply with synchronized oversampling factor
  New_Measurement : Inport  OutDataTypeStr=boolean  PortDimensions=1  SampleTime=1e-08
  rps : Inport  Port=2  OutDataTypeStr=fixdt(1, 38, 32)  PortDimensions=1  SampleTime=1e-08
  Oversampling Factor : Inport  Port=3  OutDataTypeStr=uint16  PortDimensions=1  SampleTime=1e-08
  Data Type Conversion2 : DataTypeConversion  OutDataTypeStr=fixdt(1, 24, 12)  SampleTime=1e-08  SaturateOnIntegerOverflow=off  RndMeth=Floor
  Data Type Conversion3 : DataTypeConversion  OutDataTypeStr=fixdt(0, 6, 0)  SampleTime=1e-08  SaturateOnIntegerOverflow=off  RndMeth=Floor
  Data Type Conversion4 : DataTypeConversion  OutDataTypeStr=fixdt(1, 32, 18)  SampleTime=1e-08  SaturateOnIntegerOverflow=off  RndMeth=Floor
  Div_i1 : Product  Inputs=**  OutDataTypeStr=fixdt(1, 30, 12)  SampleTime=1e-08
  Div_i1_out_dtc : DataTypeConversion  OutDataTypeStr=fixdt(1, 24, 11)  RndMeth=Simplest  SampleTime=1e-08
  HDL Reciprocal : Subsystem
  delayMatch : Delay  DelayLength=double(9)  InitialCondition=0  SampleTime=1e-08
  in_0_pipe : Delay  DelayLength=double(1)  InitialCondition=0  SampleTime=1e-08
  in_1_pipe : Delay  DelayLength=double(1)  InitialCondition=0  SampleTime=1e-08
  out_1_pipe : Delay  DelayLength=double(1)  InitialCondition=0  SampleTime=1e-08
  rd_{0..1,3..4} (4 alike) : Delay  DelayLength=double(1)  InitialCondition=0  SampleTime=1e-08
  rd_2 : Delay  DelayLength=double(8)  InitialCondition=0  SampleTime=1e-08
  omega_oversampled : Outport  SampleTime=1e-08
  New_Measurement_delayed : Outport  Port=2  SampleTime=1e-08
  wires:
  in_1_pipe/1 -> Data Type Conversion4/1
  out_1_pipe/1 -> delayMatch/1
  in_0_pipe/1 -> out_1_pipe/1
  Div_i1_out_dtc/1 -> rd_4/1
  rd_3/1 -> Div_i1_out_dtc/1
  Div_i1/1 -> rd_3/1
  rd_2/1 -> Div_i1/2
  Data Type Conversion3/1 -> rd_2/1
  Data Type Conversion2/1 -> Div_i1/1
  rd_1/1 -> Data Type Conversion3/1
  rd_0/1 -> Data Type Conversion2/1
  Oversampling Factor/1 -> rd_1/1
  rps/1 -> in_1_pipe/1
  New_Measurement/1 -> in_0_pipe/1
  HDL Reciprocal/1(Out1) -> rd_0/1
  delayMatch/1 -> New_Measurement_delayed/1
  rd_4/1 -> omega_oversampled/1
  Data Type Conversion4/1 -> HDL Reciprocal/1(In1)

== system gm_inc_enc_v25/IncEnc_V25/speed/calc_omega_instance3/invt_mult ==
  note: Invert 1/omega and muliply with synchronized oversampling factor
  New_Measurement : Inport  OutDataTypeStr=boolean  PortDimensions=1  SampleTime=1e-08
  rps : Inport  Port=2  OutDataTypeStr=fixdt(1, 38, 32)  PortDimensions=1  SampleTime=1e-08
  Oversampling Factor : Inport  Port=3  OutDataTypeStr=uint16  PortDimensions=1  SampleTime=1e-08
  Data Type Conversion2 : DataTypeConversion  OutDataTypeStr=fixdt(1, 24, 12)  SampleTime=1e-08  SaturateOnIntegerOverflow=off  RndMeth=Floor
  Data Type Conversion3 : DataTypeConversion  OutDataTypeStr=fixdt(0, 6, 0)  SampleTime=1e-08  SaturateOnIntegerOverflow=off  RndMeth=Floor
  Data Type Conversion4 : DataTypeConversion  OutDataTypeStr=fixdt(1, 32, 18)  SampleTime=1e-08  SaturateOnIntegerOverflow=off  RndMeth=Floor
  Div_i1 : Product  Inputs=**  OutDataTypeStr=fixdt(1, 30, 12)  SampleTime=1e-08
  Div_i1_out_dtc : DataTypeConversion  OutDataTypeStr=fixdt(1, 24, 11)  RndMeth=Simplest  SampleTime=1e-08
  HDL Reciprocal : Subsystem
  delayMatch : Delay  DelayLength=double(9)  InitialCondition=0  SampleTime=1e-08
  in_0_pipe : Delay  DelayLength=double(1)  InitialCondition=0  SampleTime=1e-08
  in_1_pipe : Delay  DelayLength=double(1)  InitialCondition=0  SampleTime=1e-08
  out_1_pipe : Delay  DelayLength=double(1)  InitialCondition=0  SampleTime=1e-08
  rd_{0..1,3..4} (4 alike) : Delay  DelayLength=double(1)  InitialCondition=0  SampleTime=1e-08
  rd_2 : Delay  DelayLength=double(8)  InitialCondition=0  SampleTime=1e-08
  omega_oversampled : Outport  SampleTime=1e-08
  New_Measurement_delayed : Outport  Port=2  SampleTime=1e-08
  wires:
  in_1_pipe/1 -> Data Type Conversion4/1
  out_1_pipe/1 -> delayMatch/1
  in_0_pipe/1 -> out_1_pipe/1
  Div_i1_out_dtc/1 -> rd_4/1
  rd_3/1 -> Div_i1_out_dtc/1
  Div_i1/1 -> rd_3/1
  rd_2/1 -> Div_i1/2
  Data Type Conversion3/1 -> rd_2/1
  Data Type Conversion2/1 -> Div_i1/1
  rd_1/1 -> Data Type Conversion3/1
  rd_0/1 -> Data Type Conversion2/1
  Oversampling Factor/1 -> rd_1/1
  rps/1 -> in_1_pipe/1
  New_Measurement/1 -> in_0_pipe/1
  HDL Reciprocal/1(Out1) -> rd_0/1
  delayMatch/1 -> New_Measurement_delayed/1
  rd_4/1 -> omega_oversampled/1
  Data Type Conversion4/1 -> HDL Reciprocal/1(In1)

== system gm_inc_enc_v25/IncEnc_V25/speed/calc_omega_instance4/invt_mult ==
  note: Invert 1/omega and muliply with synchronized oversampling factor
  New_Measurement : Inport  OutDataTypeStr=boolean  PortDimensions=1  SampleTime=1e-08
  rps : Inport  Port=2  OutDataTypeStr=fixdt(1, 38, 32)  PortDimensions=1  SampleTime=1e-08
  Oversampling Factor : Inport  Port=3  OutDataTypeStr=uint16  PortDimensions=1  SampleTime=1e-08
  Data Type Conversion2 : DataTypeConversion  OutDataTypeStr=fixdt(1, 24, 12)  SampleTime=1e-08  SaturateOnIntegerOverflow=off  RndMeth=Floor
  Data Type Conversion3 : DataTypeConversion  OutDataTypeStr=fixdt(0, 6, 0)  SampleTime=1e-08  SaturateOnIntegerOverflow=off  RndMeth=Floor
  Data Type Conversion4 : DataTypeConversion  OutDataTypeStr=fixdt(1, 32, 18)  SampleTime=1e-08  SaturateOnIntegerOverflow=off  RndMeth=Floor
  Div_i1 : Product  Inputs=**  OutDataTypeStr=fixdt(1, 30, 12)  SampleTime=1e-08
  Div_i1_out_dtc : DataTypeConversion  OutDataTypeStr=fixdt(1, 24, 11)  RndMeth=Simplest  SampleTime=1e-08
  HDL Reciprocal : Subsystem
  delayMatch : Delay  DelayLength=double(9)  InitialCondition=0  SampleTime=1e-08
  in_0_pipe : Delay  DelayLength=double(1)  InitialCondition=0  SampleTime=1e-08
  in_1_pipe : Delay  DelayLength=double(1)  InitialCondition=0  SampleTime=1e-08
  out_1_pipe : Delay  DelayLength=double(1)  InitialCondition=0  SampleTime=1e-08
  rd_{0..1,3..4} (4 alike) : Delay  DelayLength=double(1)  InitialCondition=0  SampleTime=1e-08
  rd_2 : Delay  DelayLength=double(8)  InitialCondition=0  SampleTime=1e-08
  omega_oversampled : Outport  SampleTime=1e-08
  New_Measurement_delayed : Outport  Port=2  SampleTime=1e-08
  wires:
  Data Type Conversion4/1 -> HDL Reciprocal/1(In1)
  rd_4/1 -> omega_oversampled/1
  delayMatch/1 -> New_Measurement_delayed/1
  HDL Reciprocal/1(Out1) -> rd_0/1
  New_Measurement/1 -> in_0_pipe/1
  rps/1 -> in_1_pipe/1
  Oversampling Factor/1 -> rd_1/1
  rd_0/1 -> Data Type Conversion2/1
  rd_1/1 -> Data Type Conversion3/1
  Data Type Conversion2/1 -> Div_i1/1
  Data Type Conversion3/1 -> rd_2/1
  rd_2/1 -> Div_i1/2
  Div_i1/1 -> rd_3/1
  rd_3/1 -> Div_i1_out_dtc/1
  Div_i1_out_dtc/1 -> rd_4/1
  in_0_pipe/1 -> out_1_pipe/1
  out_1_pipe/1 -> delayMatch/1
  in_1_pipe/1 -> Data Type Conversion4/1

== system gm_inc_enc_v25/IncEnc_V25/speed/calc_omega_instance1/invt_mult/HDL Reciprocal ==
  In1 : Inport
  Delay1 : Delay  DelayLength=1
  Delay2 : Delay  DelayLength=6
  HDL Reciprocal : Reciprocal  NumberOfIterations=reciprocal_iterations  SampleTime=1e-08
  Out1 : Outport
  wires:
  Delay2/1 -> Out1/1
  HDL Reciprocal/1 -> Delay2/1
  Delay1/1 -> HDL Reciprocal/1
  In1/1 -> Delay1/1

== system gm_inc_enc_v25/IncEnc_V25/speed/calc_omega_instance2/invt_mult/HDL Reciprocal ==
  In1 : Inport
  Delay1 : Delay  DelayLength=1
  Delay2 : Delay  DelayLength=6
  HDL Reciprocal : Reciprocal  NumberOfIterations=reciprocal_iterations  SampleTime=1e-08
  Out1 : Outport
  wires:
  Delay2/1 -> Out1/1
  HDL Reciprocal/1 -> Delay2/1
  Delay1/1 -> HDL Reciprocal/1
  In1/1 -> Delay1/1

== system gm_inc_enc_v25/IncEnc_V25/speed/calc_omega_instance3/invt_mult/HDL Reciprocal ==
  In1 : Inport
  Delay1 : Delay  DelayLength=1
  Delay2 : Delay  DelayLength=6
  HDL Reciprocal : Reciprocal  NumberOfIterations=reciprocal_iterations  SampleTime=1e-08
  Out1 : Outport
  wires:
  Delay2/1 -> Out1/1
  HDL Reciprocal/1 -> Delay2/1
  Delay1/1 -> HDL Reciprocal/1
  In1/1 -> Delay1/1

== system gm_inc_enc_v25/IncEnc_V25/speed/calc_omega_instance4/invt_mult/HDL Reciprocal ==
  In1 : Inport
  Delay1 : Delay  DelayLength=1
  Delay2 : Delay  DelayLength=6
  HDL Reciprocal : Reciprocal  NumberOfIterations=reciprocal_iterations  SampleTime=1e-08
  Out1 : Outport
  wires:
  In1/1 -> Delay1/1
  Delay1/1 -> HDL Reciprocal/1
  HDL Reciprocal/1 -> Delay2/1
  Delay2/1 -> Out1/1

== matlab function gm_inc_enc_v25/IncEnc_V25/speed/OS_factor_logic/align_oversamples/align_oversamples ==
  settings: fimath=fimath('RoundingMethod', 'Floor','OverflowAction', 'Wrap','ProductMode', 'FullPrecision', 'SumMode', 'FullPrecision')
  data: oversampling_factor input; new_transition input; states input; delay_output output
function delay_output  = fcn(oversampling_factor, new_transition, states)

% Fqint8 = fimath('RoundingMethod', 'Floor', 'OverflowAction', 'Wrap','ProductMode', 'SpecifyPrecision', 'ProductWordLength', 8,'ProductFractionLength',0,'SumMode','SpecifyPrecision','SumWordLength',8,'SumFractionLength',0);
half            = fi(0.5,false,1,1);
three_quarter   = fi(0.75,false,2,2);
persistent delay
if isempty(delay)
    delay    = logical([0 0 0 0]);
end

%% detect current ordering
if(new_transition(1) == 1) % omega_A updated
    
    %% change ordering
    %desired order when dir = +1: A, not B, not A, B => 1, 4, 3, 2
    %desired order when dir = -1: A, B, notA, not B  => 1, 2, 3, 4
    % desired order = omega1=A, omega2, omega3, omega4
    omega2= uint8(4);
    omega3= uint8(3);
    omega4= uint8(2);
    
    zero_logic = logical([0,0,0,0]);
    omega2_reset = zero_logic;
    omega3_reset = zero_logic;
    omega4_reset = zero_logic;
    
    omega2_reset(omega2) = true;
    omega3_reset(omega3) = true;
    omega4_reset(omega4) = true;
    
    omega2_target = uint8(oversampling_factor * half );
    omega3_target = uint8(oversampling_factor * three_quarter);
    omega4_target = uint8(oversampling_factor);
    
    if (oversampling_factor>=2)
        if (all(delay == 0) ) % no delay active
            
            if(states(omega4) ~= omega4_target)
                delay = omega4_reset;
                
            elseif(states(omega3) ~= omega3_target )
                delay = omega3_reset;
                
            elseif(states(omega2) ~= omega2_target )
                delay = omega2_reset;
                
            else
                delay = zero_logic; %final state is reached
            end
            
        else % a delay is already active
            if(         (delay(omega4) == 1 ) && (states(omega4) == (omega4_target-1) ) )
                delay = zero_logic;
            elseif(     (delay(omega3) == 1 ) && (states(omega3) == (omega3_target-1) ) )
                delay = zero_logic;
            %elseif(     isequal(delay, omega2_reset ) && (states(omega2) == (omega2_target-1) ) )
            elseif(     (delay(omega2) == 1 ) && (states(omega2) == (omega2_target-1) ) )
                delay = zero_logic;
            end
        end
    else
        delay = zero_logic;
    end
end

delay_output = delay;

end

== matlab function gm_inc_enc_v25/IncEnc_V25/speed/OS_factor_logic/oversample_factor/oversample_factor ==
  settings: fimath=fimath('RoundingMethod', 'Floor','OverflowAction', 'Wrap','ProductMode', 'FullPrecision', 'SumMode', 'FullPrecision')
  data: AllowCheckOverSampl input; state_Out output fixdt(0,16,0); ReadBack_Omega input; OverSamplOmega input; state input fixdt(0,16,0); InternalOmega input; InternalOmega_Out output fixdt(1,24,11)
    function [state_Out,InternalOmega_Out] = fcn(AllowCheckOverSampl, ReadBack_Omega,OverSamplOmega,state,InternalOmega)

Fq16    = fimath('RoundingMethod', 'Floor', 'OverflowAction', 'Wrap','ProductMode', 'FullPrecision', 'ProductWordLength', 16,'ProductFractionLength', 0,'SumMode','SpecifyPrecision','SumWordLength',16,'SumFractionLength',0);
Fq24    = fimath('RoundingMethod', 'Floor', 'OverflowAction', 'Wrap','ProductMode', 'FullPrecision', 'ProductWordLength', 24,'ProductFractionLength',11,'SumMode','SpecifyPrecision','SumWordLength',24,'SumFractionLength',11);

half    = fi(0.5,false,1,1);

if isempty(InternalOmega)
    InternalOmega = fi(0, 1, 24, 11);
end

%Counter State
if isempty(state)
    state = fi(1, 0, 16, 0);
end

%% Count Up 
% pre-calculate since used in comparison and assignment afterwards
Omega_ADD = fi(add(Fq24,InternalOmega,OverSamplOmega),1,24,11); 
Omega_SUB = fi(sub(Fq24,InternalOmega,OverSamplOmega),1,24,11);

if (ReadBack_Omega > Omega_ADD) && (AllowCheckOverSampl == 1)
    state= fi(add(Fq16,state,fi(1, 0, 16, 0)),0,16,0);   %Count up the measure-state
    InternalOmega = Omega_ADD;
elseif(ReadBack_Omega < Omega_SUB) && (AllowCheckOverSampl == 1)
    state= fi(sub(Fq16,state,fi(1, 0, 16, 0)),0,16,0);   %Count down the measure-state
    InternalOmega = Omega_SUB;
elseif(ReadBack_Omega < (OverSamplOmega*half)) && (AllowCheckOverSampl == 1)
    state = fi(1, 0, 16, 0);
end

%% Output the variables
state_Out = state;
InternalOmega_Out = InternalOmega;

end
